simulink model "CCModel_62"  (R2024a)
settings: Solver=ode3  StartTime=0.0  StopTime=100  FixedStep=0.001  RelTol=1e-3  EnableMultiTasking=on
undefined symbols (not defined in the file or in its folder): DiscIntNeverNeededParam, Hecate_desVel1, Hecate_desVel2, Hecate_desVel3, Hecate_horShift, Hecate_period, Hecate_slope, Hecate_Transition1, Hecate_Transition2, Hecate_verShift, i, PME_qb, qb_map, RPM_qb, V
libraries: simulink x46
(part 10 of 11)

== system CCModel_62/Powertrain/GEN/efficiency ==
  Motor speed [rpm] : Inport
  "Torque [Nm] " : Inport  Port=2
  Abs : Abs  SaturateOnIntegerOverflow=off
  Abs2 : Abs  SaturateOnIntegerOverflow=off
  Inverter efficiency : Gain  Gain=0.97
  Inverter efficiency1 : Gain  Gain=0.97
  Multiply : Gain  Gain=1/9.5488
  Product{,1..2,5} (4 alike) : Product
  Product3 : Product  Inputs=3
  Product4 : Product  Inputs=3
  RPM to rad/s : Gain  Gain=0.104719755
  RPM to rad/s1 : Gain  Gain=0.104719755
  Saturation : Saturate  UpperLimit=inf  LowerLimit=0
  Saturation1 : Saturate  UpperLimit=0  LowerLimit=-inf
  Saturation2 : Saturate  UpperLimit=inf  LowerLimit=0
  Saturation3 : Saturate  UpperLimit=inf  LowerLimit=0
  Sign : Signum  ZeroCross=off
  Subtract : Sum  Inputs=+-
  Subtract1 : Sum  Inputs=+-
  Switch : Switch  Criteria=u2 > Threshold  ZeroCross=off  SaturateOnIntegerOverflow=off  InputSameDT=off
  Terminator : Terminator
  Terminator1 : Terminator
  divider : Subsystem
  divider1 : Subsystem
  motor efficiency map : Lookup_n-D  BreakpointsForDimension1=|  BreakpointsForDimension2="[1\t440.500000000000\t881\t1321.50000000000\t1762\t2202.50000000000\t2643\t3083.50000000000\t3524\t3964.50000000000\t4405\t4845.50000000000\t5286\t5726.50000000000\t6167\t6607.50000000000\t7048\t7488.50000000000\t7929\t8369.50000000000\t8810]"  Table=|  InternalRulePriority=Speed  RndMeth=Simplest
      BreakpointsForDimension1=|
      | [1
      | 6
      | 12
      | 18
      | 36
      | 54
      | 72
      | 90
      | 108
      | 126
      | 144
      | 162
      | 180
      | 198
      | 216
      | 234
      | 252
      | 270
      | 288
      | 306
      | 324
      | 342
      | 360]
      Table=|
      | [0.100000000000000	0.100000000000000	0.420000000000000	0.440000000000000	0.450000000000000	0.460000000000000	0.470000000000000	0.480000000000000	0.490000000000000	0.500000000000000	0.510000000000000	0.520000000000000	0.530000000000000	0.540000000000000	0.550000000000000	0.560000000000000	0.580000000000000	0.560000000000000	0.550000000000000	0.540000000000000	0.500000000000000
      | 0.740000000000000	0.750000000000000	0.750000000000000	0.760000000000000	0.763000000000000	0.767000000000000	0.780000000000000	0.780000000000000	0.780000000000000	0.780000000000000	0.780000000000000	0.770000000000000	0.770000000000000	0.770000000000000	0.769000000000000	0.769000000000000	0.765000000000000	0.760000000000000	0.750000000000000	0.730000000000000	0.720000000000000
      | 0.780000000000000	0.790000000000000	0.800000000000000	0.850000000000000	0.880000000000000	0.890000000000000	0.895000000000000	0.900000000000000	0.910000000000000	0.910000000000000	0.910000000000000	0.915000000000000	0.915000000000000	0.918000000000000	0.917000000000000	0.916000000000000	0.910000000000000	0.910000000000000	0.894000000000000	0.870000000000000	0.850000000000000
      | 0.800000000000000	0.870000000000000	0.902500000000000	0.942500000000000	0.945000000000000	0.945000000000000	0.945000000000000	0.945000000000000	0.945000000000000	0.947500000000000	0.945000000000000	0.945000000000000	0.945000000000000	0.945000000000000	0.945000000000000	0.937500000000000	0.920000000000000	0.910000000000000	0.898000000000000	0.890000000000000	0.840000000000000
      | 0.800000000000000	0.880000000000000	0.902500000000000	0.947500000000000	0.953000000000000	0.955000000000000	0.957500000000000	0.957500000000000	0.956000000000000	0.960000000000000	0.960000000000000	0.960000000000000	0.960000000000000	0.957500000000000	0.957500000000000	0.955000000000000	0.950000000000000	0.945000000000000	0.940000000000000	0.920000000000000	0.890000000000000
      | 0.780000000000000	0.880000000000000	0.902500000000000	0.947500000000000	0.952500000000000	0.957500000000000	0.960000000000000	0.962000000000000	0.962500000000000	0.964000000000000	0.965000000000000	0.965000000000000	0.965000000000000	0.965000000000000	0.962500000000000	0.958000000000000	0.957000000000000	0.951000000000000	0.947500000000000	0.945000000000000	0.940000000000000
      | 0.740000000000000	0.880000000000000	0.902500000000000	0.942500000000000	0.952500000000000	0.955000000000000	0.962000000000000	0.964000000000000	0.966000000000000	0.967000000000000	0.968000000000000	0.970000000000000	0.967000000000000	0.966000000000000	0.964000000000000	0.962000000000000	0.960000000000000	0.956000000000000	0.953000000000000	0.948000000000000	0.945000000000000
      | 0.700000000000000	0.870000000000000	0.902500000000000	0.945000000000000	0.947500000000000	0.952500000000000	0.960000000000000	0.962500000000000	0.965000000000000	0.966000000000000	0.968000000000000	0.970000000000000	0.967500000000000	0.966500000000000	0.965000000000000	0.962500000000000	0.960000000000000	0.955000000000000	0.952000000000000	0.946000000000000	0.945000000000000
      | 0.650000000000000	0.860000000000000	0.902500000000000	0.932500000000000	0.942500000000000	0.950000000000000	0.957500000000000	0.961000000000000	0.963000000000000	0.965500000000000	0.967500000000000	0.970000000000000	0.967500000000000	0.965000000000000	0.964000000000000	0.960000000000000	0.957000000000000	0.953000000000000	0.950000000000000	0.945000000000000	0.942000000000000
      | 0.600000000000000	0.850000000000000	0.902500000000000	0.927500000000000	0.937500000000000	0.947500000000000	0.955000000000000	0.959000000000000	0.962500000000000	0.965000000000000	0.966000000000000	0.967500000000000	0.965000000000000	0.963000000000000	0.961800000000000	0.957500000000000	0.955000000000000	0.950000000000000	0.945000000000000	0.941000000000000	0.937500000000000
      | 0.590000000000000	0.840000000000000	0.902500000000000	0.925000000000000	0.932500000000000	0.942500000000000	0.952500000000000	0.957500000000000	0.960000000000000	0.962500000000000	0.965000000000000	0.965000000000000	0.962500000000000	0.961000000000000	0.958000000000000	0.954000000000000	0.950000000000000	0.945000000000000	0.940000000000000	0.930000000000000	0.925000000000000
      | 0.550000000000000	0.830000000000000	0.902500000000000	0.922500000000000	0.927500000000000	0.937500000000000	0.950000000000000	0.955000000000000	0.957500000000000	0.961000000000000	0.962500000000000	0.962500000000000	0.960000000000000	0.957500000000000	0.955000000000000	0.950000000000000	0.945000000000000	0.935000000000000	0.922500000000000	0.917500000000000	0.915000000000000
      | 0.540000000000000	0.820000000000000	0.890000000000000	0.920000000000000	0.922500000000000	0.935000000000000	0.947000000000000	0.952000000000000	0.955000000000000	0.958000000000000	0.961200000000000	0.960000000000000	0.957500000000000	0.954000000000000	0.950000000000000	0.942500000000000	0.932500000000000	0.922500000000000	0.912500000000000	0.910000000000000	0
      | 0.500000000000000	0.810000000000000	0.880000000000000	0.910000000000000	0.920000000000000	0.930000000000000	0.942500000000000	0.951250000000000	0.952500000000000	0.956000000000000	0.960000000000000	0.956000000000000	0.952500000000000	0.950000000000000	0.942500000000000	0.930000000000000	0.915000000000000	0.910000000000000	0	0	0
      | 0.450000000000000	0.805000000000000	0.870000000000000	0.905000000000000	0.917500000000000	0.925000000000000	0.940000000000000	0.945000000000000	0.950000000000000	0.952500000000000	0.955000000000000	0.952500000000000	0.948000000000000	0.942500000000000	0.930000000000000	0.915000000000000	0.910000000000000	0	0	0	0
      | 0.430000000000000	0.800000000000000	0.860000000000000	0.890000000000000	0.912500000000000	0.920000000000000	0.935000000000000	0.942500000000000	0.946000000000000	0.950000000000000	0.952500000000000	0.949000000000000	0.942500000000000	0.935000000000000	0.917500000000000	0.912500000000000	0	0	0	0	0
      | 0.420000000000000	0.790000000000000	0.850000000000000	0.880000000000000	0.907500000000000	0.915000000000000	0.932000000000000	0.937500000000000	0.942500000000000	0.945000000000000	0.948000000000000	0.942500000000000	0.935000000000000	0.922500000000000	0.915000000000000	0	0	0	0	0	0
      | 0.410000000000000	0.780000000000000	0.840000000000000	0.870000000000000	0.900000000000000	0.910000000000000	0.927500000000000	0.935000000000000	0.938000000000000	0.942500000000000	0.945000000000000	0.935000000000000	0.925000000000000	0.920000000000000	0	0	0	0	0	0	0
      | 0.400000000000000	0.760000000000000	0.830000000000000	0.860000000000000	0.890000000000000	0.905000000000000	0.922500000000000	0.930000000000000	0.935000000000000	0.937500000000000	0.935000000000000	0.927500000000000	0	0	0	0	0	0	0	0	0
      | 0.380000000000000	0.740000000000000	0.820000000000000	0.850000000000000	0.880000000000000	0.900000000000000	0.917500000000000	0.927500000000000	0.930000000000000	0.930000000000000	0.922500000000000	0.920000000000000	0	0	0	0	0	0	0	0	0
      | 0.360000000000000	0.710000000000000	0.810000000000000	0.840000000000000	0.875000000000000	0.897500000000000	0.912500000000000	0.922500000000000	0.925000000000000	0.928000000000000	0.915000000000000	0	0	0	0	0	0	0	0	0	0
      | 0.350000000000000	0.700000000000000	0.800000000000000	0.835000000000000	0.872500000000000	0.880000000000000	0.905000000000000	0.917500000000000	0.921000000000000	0.920000000000000	0	0	0	0	0	0	0	0	0	0	0
      | 0.350000000000000	0.680000000000000	0.790000000000000	0.830000000000000	0.870000000000000	0.875000000000000	0.900000000000000	0.910000000000000	0.900000000000000	0	0	0	0	0	0	0	0	0	0	0	0]
      settings: InputPortMap=u0,u1
  motor efficiency map1 : Lookup_n-D  BreakpointsForDimension1=|  BreakpointsForDimension2="[1\t440.500000000000\t881\t1321.50000000000\t1762\t2202.50000000000\t2643\t3083.50000000000\t3524\t3964.50000000000\t4405\t4845.50000000000\t5286\t5726.50000000000\t6167\t6607.50000000000\t7048\t7488.50000000000\t7929\t8369.50000000000\t8810]"  Table=|  InternalRulePriority=Speed  RndMeth=Simplest
      BreakpointsForDimension1=|
      | [1
      | 6
      | 12
      | 18
      | 36
      | 54
      | 72
      | 90
      | 108
      | 126
      | 144
      | 162
      | 180
      | 198
      | 216
      | 234
      | 252
      | 270
      | 288
      | 306
      | 324
      | 342
      | 360]
      Table=|
      | [0.100000000000000	0.100000000000000	0.420000000000000	0.440000000000000	0.450000000000000	0.460000000000000	0.470000000000000	0.480000000000000	0.490000000000000	0.500000000000000	0.510000000000000	0.520000000000000	0.530000000000000	0.540000000000000	0.550000000000000	0.560000000000000	0.580000000000000	0.560000000000000	0.550000000000000	0.540000000000000	0.500000000000000
      | 0.740000000000000	0.750000000000000	0.750000000000000	0.760000000000000	0.763000000000000	0.767000000000000	0.780000000000000	0.780000000000000	0.780000000000000	0.780000000000000	0.780000000000000	0.770000000000000	0.770000000000000	0.770000000000000	0.769000000000000	0.769000000000000	0.765000000000000	0.760000000000000	0.750000000000000	0.730000000000000	0.720000000000000
      | 0.780000000000000	0.790000000000000	0.800000000000000	0.850000000000000	0.880000000000000	0.890000000000000	0.895000000000000	0.900000000000000	0.910000000000000	0.910000000000000	0.910000000000000	0.915000000000000	0.915000000000000	0.918000000000000	0.917000000000000	0.916000000000000	0.910000000000000	0.910000000000000	0.894000000000000	0.870000000000000	0.850000000000000
      | 0.800000000000000	0.870000000000000	0.902500000000000	0.942500000000000	0.945000000000000	0.945000000000000	0.945000000000000	0.945000000000000	0.945000000000000	0.947500000000000	0.945000000000000	0.945000000000000	0.945000000000000	0.945000000000000	0.945000000000000	0.937500000000000	0.920000000000000	0.910000000000000	0.898000000000000	0.890000000000000	0.840000000000000
      | 0.800000000000000	0.880000000000000	0.902500000000000	0.947500000000000	0.953000000000000	0.955000000000000	0.957500000000000	0.957500000000000	0.956000000000000	0.960000000000000	0.960000000000000	0.960000000000000	0.960000000000000	0.957500000000000	0.957500000000000	0.955000000000000	0.950000000000000	0.945000000000000	0.940000000000000	0.920000000000000	0.890000000000000
      | 0.780000000000000	0.880000000000000	0.902500000000000	0.947500000000000	0.952500000000000	0.957500000000000	0.960000000000000	0.962000000000000	0.962500000000000	0.964000000000000	0.965000000000000	0.965000000000000	0.965000000000000	0.965000000000000	0.962500000000000	0.958000000000000	0.957000000000000	0.951000000000000	0.947500000000000	0.945000000000000	0.940000000000000
      | 0.740000000000000	0.880000000000000	0.902500000000000	0.942500000000000	0.952500000000000	0.955000000000000	0.962000000000000	0.964000000000000	0.966000000000000	0.967000000000000	0.968000000000000	0.970000000000000	0.967000000000000	0.966000000000000	0.964000000000000	0.962000000000000	0.960000000000000	0.956000000000000	0.953000000000000	0.948000000000000	0.945000000000000
      | 0.700000000000000	0.870000000000000	0.902500000000000	0.945000000000000	0.947500000000000	0.952500000000000	0.960000000000000	0.962500000000000	0.965000000000000	0.966000000000000	0.968000000000000	0.970000000000000	0.967500000000000	0.966500000000000	0.965000000000000	0.962500000000000	0.960000000000000	0.955000000000000	0.952000000000000	0.946000000000000	0.945000000000000
      | 0.650000000000000	0.860000000000000	0.902500000000000	0.932500000000000	0.942500000000000	0.950000000000000	0.957500000000000	0.961000000000000	0.963000000000000	0.965500000000000	0.967500000000000	0.970000000000000	0.967500000000000	0.965000000000000	0.964000000000000	0.960000000000000	0.957000000000000	0.953000000000000	0.950000000000000	0.945000000000000	0.942000000000000
      | 0.600000000000000	0.850000000000000	0.902500000000000	0.927500000000000	0.937500000000000	0.947500000000000	0.955000000000000	0.959000000000000	0.962500000000000	0.965000000000000	0.966000000000000	0.967500000000000	0.965000000000000	0.963000000000000	0.961800000000000	0.957500000000000	0.955000000000000	0.950000000000000	0.945000000000000	0.941000000000000	0.937500000000000
      | 0.590000000000000	0.840000000000000	0.902500000000000	0.925000000000000	0.932500000000000	0.942500000000000	0.952500000000000	0.957500000000000	0.960000000000000	0.962500000000000	0.965000000000000	0.965000000000000	0.962500000000000	0.961000000000000	0.958000000000000	0.954000000000000	0.950000000000000	0.945000000000000	0.940000000000000	0.930000000000000	0.925000000000000
      | 0.550000000000000	0.830000000000000	0.902500000000000	0.922500000000000	0.927500000000000	0.937500000000000	0.950000000000000	0.955000000000000	0.957500000000000	0.961000000000000	0.962500000000000	0.962500000000000	0.960000000000000	0.957500000000000	0.955000000000000	0.950000000000000	0.945000000000000	0.935000000000000	0.922500000000000	0.917500000000000	0.915000000000000
      | 0.540000000000000	0.820000000000000	0.890000000000000	0.920000000000000	0.922500000000000	0.935000000000000	0.947000000000000	0.952000000000000	0.955000000000000	0.958000000000000	0.961200000000000	0.960000000000000	0.957500000000000	0.954000000000000	0.950000000000000	0.942500000000000	0.932500000000000	0.922500000000000	0.912500000000000	0.910000000000000	0
      | 0.500000000000000	0.810000000000000	0.880000000000000	0.910000000000000	0.920000000000000	0.930000000000000	0.942500000000000	0.951250000000000	0.952500000000000	0.956000000000000	0.960000000000000	0.956000000000000	0.952500000000000	0.950000000000000	0.942500000000000	0.930000000000000	0.915000000000000	0.910000000000000	0	0	0
      | 0.450000000000000	0.805000000000000	0.870000000000000	0.905000000000000	0.917500000000000	0.925000000000000	0.940000000000000	0.945000000000000	0.950000000000000	0.952500000000000	0.955000000000000	0.952500000000000	0.948000000000000	0.942500000000000	0.930000000000000	0.915000000000000	0.910000000000000	0	0	0	0
      | 0.430000000000000	0.800000000000000	0.860000000000000	0.890000000000000	0.912500000000000	0.920000000000000	0.935000000000000	0.942500000000000	0.946000000000000	0.950000000000000	0.952500000000000	0.949000000000000	0.942500000000000	0.935000000000000	0.917500000000000	0.912500000000000	0	0	0	0	0
      | 0.420000000000000	0.790000000000000	0.850000000000000	0.880000000000000	0.907500000000000	0.915000000000000	0.932000000000000	0.937500000000000	0.942500000000000	0.945000000000000	0.948000000000000	0.942500000000000	0.935000000000000	0.922500000000000	0.915000000000000	0	0	0	0	0	0
      | 0.410000000000000	0.780000000000000	0.840000000000000	0.870000000000000	0.900000000000000	0.910000000000000	0.927500000000000	0.935000000000000	0.938000000000000	0.942500000000000	0.945000000000000	0.935000000000000	0.925000000000000	0.920000000000000	0	0	0	0	0	0	0
      | 0.400000000000000	0.760000000000000	0.830000000000000	0.860000000000000	0.890000000000000	0.905000000000000	0.922500000000000	0.930000000000000	0.935000000000000	0.937500000000000	0.935000000000000	0.927500000000000	0	0	0	0	0	0	0	0	0
      | 0.380000000000000	0.740000000000000	0.820000000000000	0.850000000000000	0.880000000000000	0.900000000000000	0.917500000000000	0.927500000000000	0.930000000000000	0.930000000000000	0.922500000000000	0.920000000000000	0	0	0	0	0	0	0	0	0
      | 0.360000000000000	0.710000000000000	0.810000000000000	0.840000000000000	0.875000000000000	0.897500000000000	0.912500000000000	0.922500000000000	0.925000000000000	0.928000000000000	0.915000000000000	0	0	0	0	0	0	0	0	0	0
      | 0.350000000000000	0.700000000000000	0.800000000000000	0.835000000000000	0.872500000000000	0.880000000000000	0.905000000000000	0.917500000000000	0.921000000000000	0.920000000000000	0	0	0	0	0	0	0	0	0	0	0
      | 0.350000000000000	0.680000000000000	0.790000000000000	0.830000000000000	0.870000000000000	0.875000000000000	0.900000000000000	0.910000000000000	0.900000000000000	0	0	0	0	0	0	0	0	0	0	0	0]
      settings: InputPortMap=u0,u1
  Electrical power [W] : Outport
  wires:
  Switch/1 -> Electrical power [W]/1  "Elec_power"
  Sign/1 -> Switch/2
  Product1/1 -> Switch/3
  divider/1(Out1) -> Switch/1
  "Torque [Nm] "/1 -> Abs/1, Product5/1, Product4/2, Abs2/1, Product3/1, Product2/2, Product/2
  Product/1 -> Multiply/1
  motor efficiency map/1 -> Saturation2/1
  motor efficiency map1/1 -> Saturation3/1
  Abs/1 -> motor efficiency map1/1
  Motor speed [rpm]/1 -> motor efficiency map1/2, RPM to rad/s1/1, Product/1, RPM to rad/s/1, motor efficiency map/2
  Saturation3/1 -> Inverter efficiency1/1
  Saturation2/1 -> Inverter efficiency/1
  Abs2/1 -> motor efficiency map/1
  RPM to rad/s/1 -> Product3/2, Product2/1
  Product3/1 -> Subtract/2
  Product2/1 -> Subtract/1
  Subtract/1 -> divider1/1(In1)
  divider1/1(Out1) -> Saturation/1  "propelling"
  RPM to rad/s1/1 -> Product5/2, Product4/3
  Product4/1 -> Subtract1/1
  Product5/1 -> Subtract1/2
  Subtract1/1 -> Saturation1/1  "ReGen"
  Multiply/1 -> Product1/1, Sign/1, divider/1(In1)  "Mech_power"
  Inverter efficiency/1 -> divider1/2(In2), Product3/3, divider/2(In2)
  Inverter efficiency1/1 -> Product4/1, Product1/2
  Saturation/1 -> Terminator/1
  Saturation1/1 -> Terminator1/1

== system CCModel_62/Powertrain/MOT/efficiency ==
  Motor speed [rpm] : Inport
  "Torque [Nm] " : Inport  Port=2
  Abs : Abs  SaturateOnIntegerOverflow=off
  Abs2 : Abs  SaturateOnIntegerOverflow=off
  Inverter efficiency : Gain  Gain=0.97
  Inverter efficiency1 : Gain  Gain=0.97
  Multiply : Gain  Gain=1/9.5488
  Product{,1..2,5} (4 alike) : Product
  Product3 : Product  Inputs=3
  Product4 : Product  Inputs=3
  RPM to rad/s : Gain  Gain=0.104719755
  RPM to rad/s1 : Gain  Gain=0.104719755
  Saturation : Saturate  UpperLimit=inf  LowerLimit=0
  Saturation1 : Saturate  UpperLimit=0  LowerLimit=-inf
  Saturation2 : Saturate  UpperLimit=inf  LowerLimit=0
  Saturation3 : Saturate  UpperLimit=inf  LowerLimit=0
  Sign : Signum  ZeroCross=off
  Subtract : Sum  Inputs=+-
  Subtract1 : Sum  Inputs=+-
  Switch : Switch  Criteria=u2 > Threshold  ZeroCross=off  SaturateOnIntegerOverflow=off  InputSameDT=off
  Terminator : Terminator
  Terminator1 : Terminator
  divider : Subsystem
  divider1 : Subsystem
  motor efficiency map : Lookup_n-D  BreakpointsForDimension1=|  BreakpointsForDimension2="[1\t440.500000000000\t881\t1321.50000000000\t1762\t2202.50000000000\t2643\t3083.50000000000\t3524\t3964.50000000000\t4405\t4845.50000000000\t5286\t5726.50000000000\t6167\t6607.50000000000\t7048\t7488.50000000000\t7929\t8369.50000000000\t8810]"  Table=|  InternalRulePriority=Speed  RndMeth=Simplest
      BreakpointsForDimension1=|
      | [1
      | 6
      | 12
      | 18
      | 36
      | 54
      | 72
      | 90
      | 108
      | 126
      | 144
      | 162
      | 180
      | 198
      | 216
      | 234
      | 252
      | 270
      | 288
      | 306
      | 324
      | 342
      | 360]
      Table=|
      | [0.100000000000000	0.100000000000000	0.420000000000000	0.440000000000000	0.450000000000000	0.460000000000000	0.470000000000000	0.480000000000000	0.490000000000000	0.500000000000000	0.510000000000000	0.520000000000000	0.530000000000000	0.540000000000000	0.550000000000000	0.560000000000000	0.580000000000000	0.560000000000000	0.550000000000000	0.540000000000000	0.500000000000000
      | 0.740000000000000	0.750000000000000	0.750000000000000	0.760000000000000	0.763000000000000	0.767000000000000	0.780000000000000	0.780000000000000	0.780000000000000	0.780000000000000	0.780000000000000	0.770000000000000	0.770000000000000	0.770000000000000	0.769000000000000	0.769000000000000	0.765000000000000	0.760000000000000	0.750000000000000	0.730000000000000	0.720000000000000
      | 0.780000000000000	0.790000000000000	0.800000000000000	0.850000000000000	0.880000000000000	0.890000000000000	0.895000000000000	0.900000000000000	0.910000000000000	0.910000000000000	0.910000000000000	0.915000000000000	0.915000000000000	0.918000000000000	0.917000000000000	0.916000000000000	0.910000000000000	0.910000000000000	0.894000000000000	0.870000000000000	0.850000000000000
      | 0.800000000000000	0.870000000000000	0.902500000000000	0.942500000000000	0.945000000000000	0.945000000000000	0.945000000000000	0.945000000000000	0.945000000000000	0.947500000000000	0.945000000000000	0.945000000000000	0.945000000000000	0.945000000000000	0.945000000000000	0.937500000000000	0.920000000000000	0.910000000000000	0.898000000000000	0.890000000000000	0.840000000000000
      | 0.800000000000000	0.880000000000000	0.902500000000000	0.947500000000000	0.953000000000000	0.955000000000000	0.957500000000000	0.957500000000000	0.956000000000000	0.960000000000000	0.960000000000000	0.960000000000000	0.960000000000000	0.957500000000000	0.957500000000000	0.955000000000000	0.950000000000000	0.945000000000000	0.940000000000000	0.920000000000000	0.890000000000000
      | 0.780000000000000	0.880000000000000	0.902500000000000	0.947500000000000	0.952500000000000	0.957500000000000	0.960000000000000	0.962000000000000	0.962500000000000	0.964000000000000	0.965000000000000	0.965000000000000	0.965000000000000	0.965000000000000	0.962500000000000	0.958000000000000	0.957000000000000	0.951000000000000	0.947500000000000	0.945000000000000	0.940000000000000
      | 0.740000000000000	0.880000000000000	0.902500000000000	0.942500000000000	0.952500000000000	0.955000000000000	0.962000000000000	0.964000000000000	0.966000000000000	0.967000000000000	0.968000000000000	0.970000000000000	0.967000000000000	0.966000000000000	0.964000000000000	0.962000000000000	0.960000000000000	0.956000000000000	0.953000000000000	0.948000000000000	0.945000000000000
      | 0.700000000000000	0.870000000000000	0.902500000000000	0.945000000000000	0.947500000000000	0.952500000000000	0.960000000000000	0.962500000000000	0.965000000000000	0.966000000000000	0.968000000000000	0.970000000000000	0.967500000000000	0.966500000000000	0.965000000000000	0.962500000000000	0.960000000000000	0.955000000000000	0.952000000000000	0.946000000000000	0.945000000000000
      | 0.650000000000000	0.860000000000000	0.902500000000000	0.932500000000000	0.942500000000000	0.950000000000000	0.957500000000000	0.961000000000000	0.963000000000000	0.965500000000000	0.967500000000000	0.970000000000000	0.967500000000000	0.965000000000000	0.964000000000000	0.960000000000000	0.957000000000000	0.953000000000000	0.950000000000000	0.945000000000000	0.942000000000000
      | 0.600000000000000	0.850000000000000	0.902500000000000	0.927500000000000	0.937500000000000	0.947500000000000	0.955000000000000	0.959000000000000	0.962500000000000	0.965000000000000	0.966000000000000	0.967500000000000	0.965000000000000	0.963000000000000	0.961800000000000	0.957500000000000	0.955000000000000	0.950000000000000	0.945000000000000	0.941000000000000	0.937500000000000
      | 0.590000000000000	0.840000000000000	0.902500000000000	0.925000000000000	0.932500000000000	0.942500000000000	0.952500000000000	0.957500000000000	0.960000000000000	0.962500000000000	0.965000000000000	0.965000000000000	0.962500000000000	0.961000000000000	0.958000000000000	0.954000000000000	0.950000000000000	0.945000000000000	0.940000000000000	0.930000000000000	0.925000000000000
      | 0.550000000000000	0.830000000000000	0.902500000000000	0.922500000000000	0.927500000000000	0.937500000000000	0.950000000000000	0.955000000000000	0.957500000000000	0.961000000000000	0.962500000000000	0.962500000000000	0.960000000000000	0.957500000000000	0.955000000000000	0.950000000000000	0.945000000000000	0.935000000000000	0.922500000000000	0.917500000000000	0.915000000000000
      | 0.540000000000000	0.820000000000000	0.890000000000000	0.920000000000000	0.922500000000000	0.935000000000000	0.947000000000000	0.952000000000000	0.955000000000000	0.958000000000000	0.961200000000000	0.960000000000000	0.957500000000000	0.954000000000000	0.950000000000000	0.942500000000000	0.932500000000000	0.922500000000000	0.912500000000000	0.910000000000000	0
      | 0.500000000000000	0.810000000000000	0.880000000000000	0.910000000000000	0.920000000000000	0.930000000000000	0.942500000000000	0.951250000000000	0.952500000000000	0.956000000000000	0.960000000000000	0.956000000000000	0.952500000000000	0.950000000000000	0.942500000000000	0.930000000000000	0.915000000000000	0.910000000000000	0	0	0
      | 0.450000000000000	0.805000000000000	0.870000000000000	0.905000000000000	0.917500000000000	0.925000000000000	0.940000000000000	0.945000000000000	0.950000000000000	0.952500000000000	0.955000000000000	0.952500000000000	0.948000000000000	0.942500000000000	0.930000000000000	0.915000000000000	0.910000000000000	0	0	0	0
      | 0.430000000000000	0.800000000000000	0.860000000000000	0.890000000000000	0.912500000000000	0.920000000000000	0.935000000000000	0.942500000000000	0.946000000000000	0.950000000000000	0.952500000000000	0.949000000000000	0.942500000000000	0.935000000000000	0.917500000000000	0.912500000000000	0	0	0	0	0
      | 0.420000000000000	0.790000000000000	0.850000000000000	0.880000000000000	0.907500000000000	0.915000000000000	0.932000000000000	0.937500000000000	0.942500000000000	0.945000000000000	0.948000000000000	0.942500000000000	0.935000000000000	0.922500000000000	0.915000000000000	0	0	0	0	0	0
      | 0.410000000000000	0.780000000000000	0.840000000000000	0.870000000000000	0.900000000000000	0.910000000000000	0.927500000000000	0.935000000000000	0.938000000000000	0.942500000000000	0.945000000000000	0.935000000000000	0.925000000000000	0.920000000000000	0	0	0	0	0	0	0
      | 0.400000000000000	0.760000000000000	0.830000000000000	0.860000000000000	0.890000000000000	0.905000000000000	0.922500000000000	0.930000000000000	0.935000000000000	0.937500000000000	0.935000000000000	0.927500000000000	0	0	0	0	0	0	0	0	0
      | 0.380000000000000	0.740000000000000	0.820000000000000	0.850000000000000	0.880000000000000	0.900000000000000	0.917500000000000	0.927500000000000	0.930000000000000	0.930000000000000	0.922500000000000	0.920000000000000	0	0	0	0	0	0	0	0	0
      | 0.360000000000000	0.710000000000000	0.810000000000000	0.840000000000000	0.875000000000000	0.897500000000000	0.912500000000000	0.922500000000000	0.925000000000000	0.928000000000000	0.915000000000000	0	0	0	0	0	0	0	0	0	0
      | 0.350000000000000	0.700000000000000	0.800000000000000	0.835000000000000	0.872500000000000	0.880000000000000	0.905000000000000	0.917500000000000	0.921000000000000	0.920000000000000	0	0	0	0	0	0	0	0	0	0	0
      | 0.350000000000000	0.680000000000000	0.790000000000000	0.830000000000000	0.870000000000000	0.875000000000000	0.900000000000000	0.910000000000000	0.900000000000000	0	0	0	0	0	0	0	0	0	0	0	0]
      settings: InputPortMap=u0,u1
  motor efficiency map1 : Lookup_n-D  BreakpointsForDimension1=|  BreakpointsForDimension2="[1\t440.500000000000\t881\t1321.50000000000\t1762\t2202.50000000000\t2643\t3083.50000000000\t3524\t3964.50000000000\t4405\t4845.50000000000\t5286\t5726.50000000000\t6167\t6607.50000000000\t7048\t7488.50000000000\t7929\t8369.50000000000\t8810]"  Table=|  InternalRulePriority=Speed  RndMeth=Simplest
      BreakpointsForDimension1=|
      | [1
      | 6
      | 12
      | 18
      | 36
      | 54
      | 72
      | 90
      | 108
      | 126
      | 144
      | 162
      | 180
      | 198
      | 216
      | 234
      | 252
      | 270
      | 288
      | 306
      | 324
      | 342
      | 360]
      Table=|
      | [0.100000000000000	0.100000000000000	0.420000000000000	0.440000000000000	0.450000000000000	0.460000000000000	0.470000000000000	0.480000000000000	0.490000000000000	0.500000000000000	0.510000000000000	0.520000000000000	0.530000000000000	0.540000000000000	0.550000000000000	0.560000000000000	0.580000000000000	0.560000000000000	0.550000000000000	0.540000000000000	0.500000000000000
      | 0.740000000000000	0.750000000000000	0.750000000000000	0.760000000000000	0.763000000000000	0.767000000000000	0.780000000000000	0.780000000000000	0.780000000000000	0.780000000000000	0.780000000000000	0.770000000000000	0.770000000000000	0.770000000000000	0.769000000000000	0.769000000000000	0.765000000000000	0.760000000000000	0.750000000000000	0.730000000000000	0.720000000000000
      | 0.780000000000000	0.790000000000000	0.800000000000000	0.850000000000000	0.880000000000000	0.890000000000000	0.895000000000000	0.900000000000000	0.910000000000000	0.910000000000000	0.910000000000000	0.915000000000000	0.915000000000000	0.918000000000000	0.917000000000000	0.916000000000000	0.910000000000000	0.910000000000000	0.894000000000000	0.870000000000000	0.850000000000000
      | 0.800000000000000	0.870000000000000	0.902500000000000	0.942500000000000	0.945000000000000	0.945000000000000	0.945000000000000	0.945000000000000	0.945000000000000	0.947500000000000	0.945000000000000	0.945000000000000	0.945000000000000	0.945000000000000	0.945000000000000	0.937500000000000	0.920000000000000	0.910000000000000	0.898000000000000	0.890000000000000	0.840000000000000
      | 0.800000000000000	0.880000000000000	0.902500000000000	0.947500000000000	0.953000000000000	0.955000000000000	0.957500000000000	0.957500000000000	0.956000000000000	0.960000000000000	0.960000000000000	0.960000000000000	0.960000000000000	0.957500000000000	0.957500000000000	0.955000000000000	0.950000000000000	0.945000000000000	0.940000000000000	0.920000000000000	0.890000000000000
      | 0.780000000000000	0.880000000000000	0.902500000000000	0.947500000000000	0.952500000000000	0.957500000000000	0.960000000000000	0.962000000000000	0.962500000000000	0.964000000000000	0.965000000000000	0.965000000000000	0.965000000000000	0.965000000000000	0.962500000000000	0.958000000000000	0.957000000000000	0.951000000000000	0.947500000000000	0.945000000000000	0.940000000000000
      | 0.740000000000000	0.880000000000000	0.902500000000000	0.942500000000000	0.952500000000000	0.955000000000000	0.962000000000000	0.964000000000000	0.966000000000000	0.967000000000000	0.968000000000000	0.970000000000000	0.967000000000000	0.966000000000000	0.964000000000000	0.962000000000000	0.960000000000000	0.956000000000000	0.953000000000000	0.948000000000000	0.945000000000000
      | 0.700000000000000	0.870000000000000	0.902500000000000	0.945000000000000	0.947500000000000	0.952500000000000	0.960000000000000	0.962500000000000	0.965000000000000	0.966000000000000	0.968000000000000	0.970000000000000	0.967500000000000	0.966500000000000	0.965000000000000	0.962500000000000	0.960000000000000	0.955000000000000	0.952000000000000	0.946000000000000	0.945000000000000
      | 0.650000000000000	0.860000000000000	0.902500000000000	0.932500000000000	0.942500000000000	0.950000000000000	0.957500000000000	0.961000000000000	0.963000000000000	0.965500000000000	0.967500000000000	0.970000000000000	0.967500000000000	0.965000000000000	0.964000000000000	0.960000000000000	0.957000000000000	0.953000000000000	0.950000000000000	0.945000000000000	0.942000000000000
      | 0.600000000000000	0.850000000000000	0.902500000000000	0.927500000000000	0.937500000000000	0.947500000000000	0.955000000000000	0.959000000000000	0.962500000000000	0.965000000000000	0.966000000000000	0.967500000000000	0.965000000000000	0.963000000000000	0.961800000000000	0.957500000000000	0.955000000000000	0.950000000000000	0.945000000000000	0.941000000000000	0.937500000000000
      | 0.590000000000000	0.840000000000000	0.902500000000000	0.925000000000000	0.932500000000000	0.942500000000000	0.952500000000000	0.957500000000000	0.960000000000000	0.962500000000000	0.965000000000000	0.965000000000000	0.962500000000000	0.961000000000000	0.958000000000000	0.954000000000000	0.950000000000000	0.945000000000000	0.940000000000000	0.930000000000000	0.925000000000000
      | 0.550000000000000	0.830000000000000	0.902500000000000	0.922500000000000	0.927500000000000	0.937500000000000	0.950000000000000	0.955000000000000	0.957500000000000	0.961000000000000	0.962500000000000	0.962500000000000	0.960000000000000	0.957500000000000	0.955000000000000	0.950000000000000	0.945000000000000	0.935000000000000	0.922500000000000	0.917500000000000	0.915000000000000
      | 0.540000000000000	0.820000000000000	0.890000000000000	0.920000000000000	0.922500000000000	0.935000000000000	0.947000000000000	0.952000000000000	0.955000000000000	0.958000000000000	0.961200000000000	0.960000000000000	0.957500000000000	0.954000000000000	0.950000000000000	0.942500000000000	0.932500000000000	0.922500000000000	0.912500000000000	0.910000000000000	0
      | 0.500000000000000	0.810000000000000	0.880000000000000	0.910000000000000	0.920000000000000	0.930000000000000	0.942500000000000	0.951250000000000	0.952500000000000	0.956000000000000	0.960000000000000	0.956000000000000	0.952500000000000	0.950000000000000	0.942500000000000	0.930000000000000	0.915000000000000	0.910000000000000	0	0	0
      | 0.450000000000000	0.805000000000000	0.870000000000000	0.905000000000000	0.917500000000000	0.925000000000000	0.940000000000000	0.945000000000000	0.950000000000000	0.952500000000000	0.955000000000000	0.952500000000000	0.948000000000000	0.942500000000000	0.930000000000000	0.915000000000000	0.910000000000000	0	0	0	0
      | 0.430000000000000	0.800000000000000	0.860000000000000	0.890000000000000	0.912500000000000	0.920000000000000	0.935000000000000	0.942500000000000	0.946000000000000	0.950000000000000	0.952500000000000	0.949000000000000	0.942500000000000	0.935000000000000	0.917500000000000	0.912500000000000	0	0	0	0	0
      | 0.420000000000000	0.790000000000000	0.850000000000000	0.880000000000000	0.907500000000000	0.915000000000000	0.932000000000000	0.937500000000000	0.942500000000000	0.945000000000000	0.948000000000000	0.942500000000000	0.935000000000000	0.922500000000000	0.915000000000000	0	0	0	0	0	0
      | 0.410000000000000	0.780000000000000	0.840000000000000	0.870000000000000	0.900000000000000	0.910000000000000	0.927500000000000	0.935000000000000	0.938000000000000	0.942500000000000	0.945000000000000	0.935000000000000	0.925000000000000	0.920000000000000	0	0	0	0	0	0	0
      | 0.400000000000000	0.760000000000000	0.830000000000000	0.860000000000000	0.890000000000000	0.905000000000000	0.922500000000000	0.930000000000000	0.935000000000000	0.937500000000000	0.935000000000000	0.927500000000000	0	0	0	0	0	0	0	0	0
      | 0.380000000000000	0.740000000000000	0.820000000000000	0.850000000000000	0.880000000000000	0.900000000000000	0.917500000000000	0.927500000000000	0.930000000000000	0.930000000000000	0.922500000000000	0.920000000000000	0	0	0	0	0	0	0	0	0
      | 0.360000000000000	0.710000000000000	0.810000000000000	0.840000000000000	0.875000000000000	0.897500000000000	0.912500000000000	0.922500000000000	0.925000000000000	0.928000000000000	0.915000000000000	0	0	0	0	0	0	0	0	0	0
      | 0.350000000000000	0.700000000000000	0.800000000000000	0.835000000000000	0.872500000000000	0.880000000000000	0.905000000000000	0.917500000000000	0.921000000000000	0.920000000000000	0	0	0	0	0	0	0	0	0	0	0
      | 0.350000000000000	0.680000000000000	0.790000000000000	0.830000000000000	0.870000000000000	0.875000000000000	0.900000000000000	0.910000000000000	0.900000000000000	0	0	0	0	0	0	0	0	0	0	0	0]
      settings: InputPortMap=u0,u1
  Electrical power [W] : Outport
  wires:
  Switch/1 -> Electrical power [W]/1  "Elec_power"
  Sign/1 -> Switch/2
  Product1/1 -> Switch/3
  divider/1(Out1) -> Switch/1
  "Torque [Nm] "/1 -> Abs/1, Product5/1, Product4/2, Abs2/1, Product3/1, Product2/2, Product/2
  Product/1 -> Multiply/1
  motor efficiency map/1 -> Saturation2/1
  motor efficiency map1/1 -> Saturation3/1
  Abs/1 -> motor efficiency map1/1
  Motor speed [rpm]/1 -> motor efficiency map1/2, RPM to rad/s1/1, Product/1, RPM to rad/s/1, motor efficiency map/2
  Saturation3/1 -> Inverter efficiency1/1
  Saturation2/1 -> Inverter efficiency/1
  Abs2/1 -> motor efficiency map/1
  RPM to rad/s/1 -> Product3/2, Product2/1
  Product3/1 -> Subtract/2
  Product2/1 -> Subtract/1
  Subtract/1 -> divider1/1(In1)
  divider1/1(Out1) -> Saturation/1  "propelling"
  RPM to rad/s1/1 -> Product5/2, Product4/3
  Product4/1 -> Subtract1/1
  Product5/1 -> Subtract1/2
  Subtract1/1 -> Saturation1/1  "ReGen"
  Multiply/1 -> Product1/1, Sign/1, divider/1(In1)  "Mech_power"
  Inverter efficiency/1 -> divider1/2(In2), Product3/3, divider/2(In2)
  Inverter efficiency1/1 -> Product4/1, Product1/2
  Saturation/1 -> Terminator/1
  Saturation1/1 -> Terminator1/1

== system CCModel_62/Powertrain/Rear Differential/Limited Slip Diff ==
  diff center front output shaft torque : Inport
  wheel front right omega : Inport  Port=2
  wheel front left omega : Inport  Port=3
  " " : Memory
  "   " : Memory
  "    " : Memory
  "       " : Memory
  "          " : Math  Operator=pow  SignedPower=on
  AbsDeltaOmega : Abs  SaturateOnIntegerOverflow=off
  AbsT : Abs  SaturateOnIntegerOverflow=off
  C0 : Constant  Value=C0
  C1 : Gain  Gain=C1
  C2 : Gain  Gain=C2
  C3 : Constant  Value=C3
  C4 : Gain  Gain=-1
  DeltaTorqueL : Product  Inputs=**
  DeltaTorqueR : Product  Inputs=**
  Sign : Lookup  InputValues=[-1000 -100 -1 -0.5 0 .5 1 100 1000]  Table=[-1 -1 -1 0 0 0 1 1 1]  SaturateOnIntegerOverflow=off
  Sum : Sum  Inputs=+-
  Sum3 : Sum  Inputs=+++  SaturateOnIntegerOverflow=on
  wheel front left torque : Outport
  wheel front right torque : Outport  Port=2
  wires:
  C0/1 -> Sum3/1
  C2/1 -> "          "/1
  "    "/1 -> DeltaTorqueL/2, DeltaTorqueR/2
  "       "/1 -> Sum3/3
  DeltaTorqueR/1 -> C4/1
  Sign/1 -> "    "/1
  C1/1 -> Sum3/2
  Sum3/1 -> DeltaTorqueR/1, DeltaTorqueL/1
  C4/1 -> wheel front right torque/1
  AbsT/1 -> "   "/1
  "          "/1 -> "       "/1
  AbsDeltaOmega/1 -> " "/1
  wheel front left omega/1 -> Sum/2
  "   "/1 -> C1/1
  diff center front output shaft torque/1 -> AbsT/1
  " "/1 -> C2/1
  DeltaTorqueL/1 -> wheel front left torque/1
  C3/1 -> "          "/2
  Sum/1 -> Sign/1, AbsDeltaOmega/1
  wheel front right omega/1 -> Sum/1

== system CCModel_62/Cruise Control/Version 4.0/Switches/Sigmoid_brake ==
  Change_time : Inport
  Old brake : Inport  Port=2
  New brake : Inport  Port=3
  Add : Sum
  Add1 : Sum
  Add2 : Sum
  Clock : Clock
  Constant : Constant
  Constant1 : Constant
  Constant2 : Constant
  Divide : Product  Inputs=/*
  Divide1 : Product  Inputs=**
  Divide2 : Product  Inputs=/*
  Divide3 : Product  Inputs=**
  Gain : Gain  Gain=1000
  Gain1 : Gain  Gain=0.001
  K : Constant
  Power{,1..3} (4 alike) : Math  Operator=pow
  Reciprocal : Product  Inputs=/
  Reciprocal1 : Product  Inputs=/
  Round : Rounding  Operator=round
  Scope : Scope  NumInputPorts=3
  Subtract : Sum  Inputs=-+
  Sum : Sum  Inputs=|-+
  brake_out : Outport
  wires:
  Power1/1 -> Scope/3, Add/1
  Add/1 -> Power/1
  Clock/1 -> Sum/2
  Constant/1 -> Add/2
  Sum/1 -> Gain/1  "Elapsed Time"
  Reciprocal/1 -> Power/2
  Power/1 -> Divide/1
  Divide/1 -> Divide1/1  "Sigmoid Function"
  Add1/1 -> Power2/1
  Power3/1 -> Add1/1
  K/1 -> Scope/2, Reciprocal/1, Power1/2, Reciprocal1/1, Power3/2
  Reciprocal1/1 -> Power2/2
  Power2/1 -> Divide2/1
  Constant1/1 -> Add1/2
  Change_time/1 -> Sum/1
  Constant2/1 -> Subtract/2
  Divide2/1 -> Subtract/1  "Sigmoid Function"
  Divide1/1 -> Add2/1
  Add2/1 -> brake_out/1
  New brake/1 -> Divide1/2
  Old brake/1 -> Divide3/2
  Subtract/1 -> Divide3/1
  Divide3/1 -> Add2/2
  Gain1/1 -> Power1/1, Divide/2, Scope/1, Divide2/2, Power3/1
  Gain/1 -> Round/1
  Round/1 -> Gain1/1

== system CCModel_62/Cruise Control/Version 4.0/Switches/Sigmoid_throttle ==
  Change_time : Inport
  Old thr : Inport  Port=2
  New thr : Inport  Port=3
  Add : Sum
  Add1 : Sum
  Add2 : Sum
  Clock : Clock
  Constant : Constant
  Constant1 : Constant
  Constant2 : Constant
  Divide : Product  Inputs=/*
  Divide1 : Product  Inputs=**
  Divide2 : Product  Inputs=/*
  Divide3 : Product  Inputs=**
  Gain : Gain  Gain=1000
  Gain1 : Gain  Gain=0.001
  K : Constant  Value=1.5
  Power{,1..3} (4 alike) : Math  Operator=pow
  Reciprocal : Product  Inputs=/
  Reciprocal1 : Product  Inputs=/
  Round : Rounding  Operator=round
  Scope : Scope  NumInputPorts=3
  Subtract : Sum  Inputs=-+
  Sum : Sum  Inputs=|-+
  throttle_out : Outport
  wires:
  Power1/1 -> Scope/3, Add/1
  Add/1 -> Power/1
  Clock/1 -> Sum/2
  Constant/1 -> Add/2
  Sum/1 -> Gain/1  "Elapsed Time"
  Reciprocal/1 -> Power/2
  Power/1 -> Divide/1
  Divide/1 -> Divide1/1  "Sigmoid Function"
  Add1/1 -> Power2/1
  Power3/1 -> Add1/1
  K/1 -> Scope/2, Reciprocal/1, Power1/2, Reciprocal1/1, Power3/2
  Reciprocal1/1 -> Power2/2
  Power2/1 -> Divide2/1
  Constant1/1 -> Add1/2
  Change_time/1 -> Sum/1
  Constant2/1 -> Subtract/2
  Divide2/1 -> Subtract/1  "Sigmoid Function"
  Divide1/1 -> Add2/1
  Add2/1 -> throttle_out/1
  New thr/1 -> Divide1/2
  Old thr/1 -> Divide3/2
  Subtract/1 -> Divide3/1
  Divide3/1 -> Add2/2
  Gain1/1 -> Power1/1, Divide/2, Scope/1, Divide2/2, Power3/1
  Gain/1 -> Round/1
  Round/1 -> Gain1/1

== system CCModel_62/Cruise Control/Version 5.0/Switches/Sigmoid_brake ==
  Change_time : Inport
  Old brake : Inport  Port=2
  New brake : Inport  Port=3
  Add : Sum
  Add1 : Sum
  Add2 : Sum
  Clock : Clock
  Constant : Constant
  Constant1 : Constant
  Constant2 : Constant
  Divide : Product  Inputs=/*
  Divide1 : Product  Inputs=**
  Divide2 : Product  Inputs=/*
  Divide3 : Product  Inputs=**
  Gain : Gain  Gain=1000
  Gain1 : Gain  Gain=0.001
  K : Constant
  Power{,1..3} (4 alike) : Math  Operator=pow
  Reciprocal : Product  Inputs=/
  Reciprocal1 : Product  Inputs=/
  Round : Rounding  Operator=round
  Scope : Scope  NumInputPorts=3
  Subtract : Sum  Inputs=-+
  Sum : Sum  Inputs=|-+
  brake_out : Outport
  wires:
  Power1/1 -> Scope/3, Add/1
  Add/1 -> Power/1
  Clock/1 -> Sum/2
  Constant/1 -> Add/2
  Sum/1 -> Gain/1  "Elapsed Time"
  Reciprocal/1 -> Power/2
  Power/1 -> Divide/1
  Divide/1 -> Divide1/1  "Sigmoid Function"
  Add1/1 -> Power2/1
  Power3/1 -> Add1/1
  K/1 -> Scope/2, Reciprocal/1, Power1/2, Reciprocal1/1, Power3/2
  Reciprocal1/1 -> Power2/2
  Power2/1 -> Divide2/1
  Constant1/1 -> Add1/2
  Change_time/1 -> Sum/1
  Constant2/1 -> Subtract/2
  Divide2/1 -> Subtract/1  "Sigmoid Function"
  Divide1/1 -> Add2/1
  Add2/1 -> brake_out/1
  New brake/1 -> Divide1/2
  Old brake/1 -> Divide3/2
  Subtract/1 -> Divide3/1
  Divide3/1 -> Add2/2
  Gain1/1 -> Power1/1, Divide/2, Scope/1, Divide2/2, Power3/1
  Gain/1 -> Round/1
  Round/1 -> Gain1/1

== system CCModel_62/Cruise Control/Version 5.0/Switches/Sigmoid_throttle ==
  Change_time : Inport
  Old thr : Inport  Port=2
  New thr : Inport  Port=3
  Add : Sum
  Add1 : Sum
  Add2 : Sum
  Clock : Clock
  Constant : Constant
  Constant1 : Constant
  Constant2 : Constant
  Divide : Product  Inputs=/*
  Divide1 : Product  Inputs=**
  Divide2 : Product  Inputs=/*
  Divide3 : Product  Inputs=**
  Gain : Gain  Gain=1000
  Gain1 : Gain  Gain=0.001
  K : Constant  Value=1.5
  Power{,1..3} (4 alike) : Math  Operator=pow
  Reciprocal : Product  Inputs=/
  Reciprocal1 : Product  Inputs=/
  Round : Rounding  Operator=round
  Scope : Scope  NumInputPorts=3
  Subtract : Sum  Inputs=-+
  Sum : Sum  Inputs=|-+
  throttle_out : Outport
  wires:
  Power1/1 -> Scope/3, Add/1
  Add/1 -> Power/1
  Clock/1 -> Sum/2
  Constant/1 -> Add/2
  Sum/1 -> Gain/1  "Elapsed Time"
  Reciprocal/1 -> Power/2
  Power/1 -> Divide/1
  Divide/1 -> Divide1/1  "Sigmoid Function"
  Add1/1 -> Power2/1
  Power3/1 -> Add1/1
  K/1 -> Scope/2, Reciprocal/1, Power1/2, Reciprocal1/1, Power3/2
  Reciprocal1/1 -> Power2/2
  Power2/1 -> Divide2/1
  Constant1/1 -> Add1/2
  Change_time/1 -> Sum/1
  Constant2/1 -> Subtract/2
  Divide2/1 -> Subtract/1  "Sigmoid Function"
  Divide1/1 -> Add2/1
  Add2/1 -> throttle_out/1
  New thr/1 -> Divide1/2
  Old thr/1 -> Divide3/2
  Subtract/1 -> Divide3/1
  Divide3/1 -> Add2/2
  Gain1/1 -> Power1/1, Divide/2, Scope/1, Divide2/2, Power3/1
  Gain/1 -> Round/1
  Round/1 -> Gain1/1

== system CCModel_62/Cruise Control/Version 6.0/Switches/Sigmoid_brake ==
  Change_time : Inport
  Old brake : Inport  Port=2
  New brake : Inport  Port=3
  Add : Sum
  Add1 : Sum
  Add2 : Sum
  Clock : Clock
  Constant : Constant
  Constant1 : Constant
  Constant2 : Constant
  Divide : Product  Inputs=/*
  Divide1 : Product  Inputs=**
  Divide2 : Product  Inputs=/*
  Divide3 : Product  Inputs=**
  Gain : Gain  Gain=1000
  Gain1 : Gain  Gain=0.001
  K : Constant
  Power{,1..3} (4 alike) : Math  Operator=pow
  Reciprocal : Product  Inputs=/
  Reciprocal1 : Product  Inputs=/
  Round : Rounding  Operator=round
  Scope : Scope  NumInputPorts=3
  Subtract : Sum  Inputs=-+
  Sum : Sum  Inputs=|-+
  brake_out : Outport
  wires:
  Power1/1 -> Scope/3, Add/1
  Add/1 -> Power/1
  Clock/1 -> Sum/2
  Constant/1 -> Add/2
  Sum/1 -> Gain/1  "Elapsed Time"
  Reciprocal/1 -> Power/2
  Power/1 -> Divide/1
  Divide/1 -> Divide1/1  "Sigmoid Function"
  Add1/1 -> Power2/1
  Power3/1 -> Add1/1
  K/1 -> Scope/2, Reciprocal/1, Power1/2, Reciprocal1/1, Power3/2
  Reciprocal1/1 -> Power2/2
  Power2/1 -> Divide2/1
  Constant1/1 -> Add1/2
  Change_time/1 -> Sum/1
  Constant2/1 -> Subtract/2
  Divide2/1 -> Subtract/1  "Sigmoid Function"
  Divide1/1 -> Add2/1
  Add2/1 -> brake_out/1
  New brake/1 -> Divide1/2
  Old brake/1 -> Divide3/2
  Subtract/1 -> Divide3/1
  Divide3/1 -> Add2/2
  Gain1/1 -> Power1/1, Divide/2, Scope/1, Divide2/2, Power3/1
  Gain/1 -> Round/1
  Round/1 -> Gain1/1

== system CCModel_62/Cruise Control/Version 6.0/Switches/Sigmoid_throttle ==
  Change_time : Inport
  Old thr : Inport  Port=2
  New thr : Inport  Port=3
  Add : Sum
  Add1 : Sum
  Add2 : Sum
  Clock : Clock
  Constant : Constant
  Constant1 : Constant
  Constant2 : Constant
  Divide : Product  Inputs=/*
  Divide1 : Product  Inputs=**
  Divide2 : Product  Inputs=/*
  Divide3 : Product  Inputs=**
  Gain : Gain  Gain=1000
  Gain1 : Gain  Gain=0.001
  K : Constant  Value=1.5
  Power{,1..3} (4 alike) : Math  Operator=pow
  Reciprocal : Product  Inputs=/
  Reciprocal1 : Product  Inputs=/
  Round : Rounding  Operator=round
  Scope : Scope  NumInputPorts=3
  Subtract : Sum  Inputs=-+
  Sum : Sum  Inputs=|-+
  throttle_out : Outport
  wires:
  Power1/1 -> Scope/3, Add/1
  Add/1 -> Power/1
  Clock/1 -> Sum/2
  Constant/1 -> Add/2
  Sum/1 -> Gain/1  "Elapsed Time"
  Reciprocal/1 -> Power/2
  Power/1 -> Divide/1
  Divide/1 -> Divide1/1  "Sigmoid Function"
  Add1/1 -> Power2/1
  Power3/1 -> Add1/1
  K/1 -> Scope/2, Reciprocal/1, Power1/2, Reciprocal1/1, Power3/2
  Reciprocal1/1 -> Power2/2
  Power2/1 -> Divide2/1
  Constant1/1 -> Add1/2
  Change_time/1 -> Sum/1
  Constant2/1 -> Subtract/2
  Divide2/1 -> Subtract/1  "Sigmoid Function"
  Divide1/1 -> Add2/1
  Add2/1 -> throttle_out/1
  New thr/1 -> Divide1/2
  Old thr/1 -> Divide3/2
  Subtract/1 -> Divide3/1
  Divide3/1 -> Add2/2
  Gain1/1 -> Power1/1, Divide/2, Scope/1, Divide2/2, Power3/1
  Gain/1 -> Round/1
  Round/1 -> Gain1/1
